simulink model "prueba_flujocarga_10_dic"  (R2015a)
settings: Solver=ode45  StartTime=0.0  StopTime=0.32  RelTol=1e-3
libraries: powerlib x31, powerlib_meascontrol x1
settings Model: Creator=USUARIO  LastModifiedBy=USUARIO

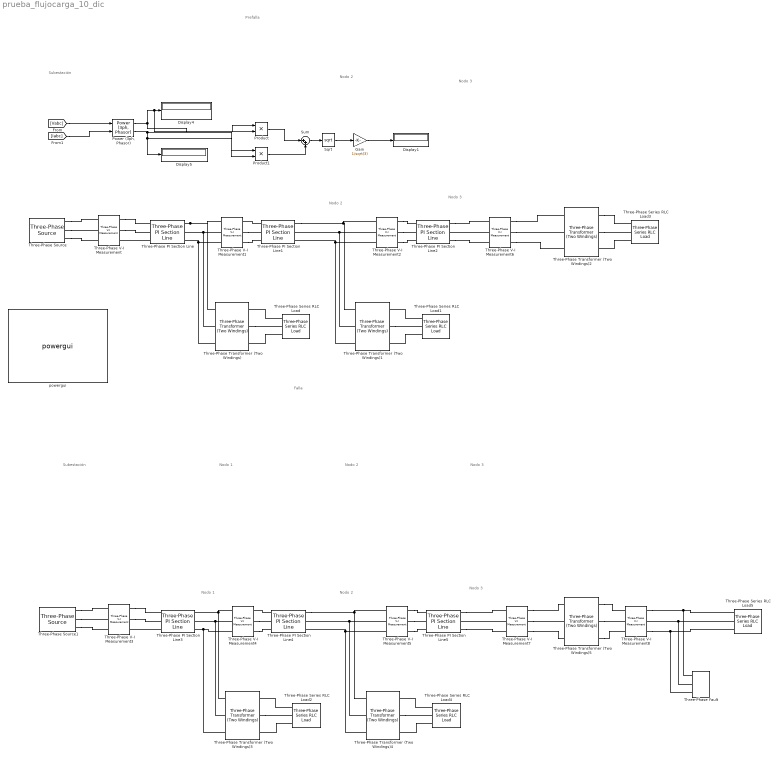
== system prueba_flujocarga_10_dic ==
  note: Falla
  note: Prefalla
  note: Nodo 2
  note: Subestación
  note: Nodo 2
  note: Nodo 1
  note: Nodo 1
  note: Nodo 2
  note: Subestación
  note: Nodo 2
  note: Nodo 3
  note: Nodo 3
  note: Nodo 3
  note: Nodo 3
  Display1 : Display
  Display4 : Display
  Display5 : Display
  Gain : Gain  Gain=1/sqrt(3)
  "Power (3ph, Phasor)" : powerlib_meascontrol/Measurements/Power (3ph, Phasor)
  Product : Product
  Product1 : Product
  Sqrt : Sqrt  SaturateOnIntegerOverflow=on
  Sum : Sum  Inputs=|++
  Three-Phase PI Section Line : powerlib/Elements/Three-Phase PI Section Line  LConnTagsString=a|b|c  RConnTagsString=A|B|C  Frequency=60  Resistances=[ 0.01273 0.3864]  Inductances="[ 0.9337e-3  4.1264e-3]"  Capacitances=[12.74e-9 7.751e-9]  Length=2
  Three-Phase PI Section Line1 : powerlib/Elements/Three-Phase PI Section Line  LConnTagsString=a|b|c  RConnTagsString=A|B|C  Frequency=60  Resistances=[ 0.01273 0.3864]  Inductances="[ 0.9337e-3  4.1264e-3]"  Capacitances=[12.74e-9 7.751e-9]  Length=1
  Three-Phase PI Section Line2 : powerlib/Elements/Three-Phase PI Section Line  LConnTagsString=a|b|c  RConnTagsString=A|B|C  Frequency=60  Resistances=[ 0.01273 0.3864]  Inductances="[ 0.9337e-3  4.1264e-3]"  Capacitances=[12.74e-9 7.751e-9]  Length=1.5
  Three-Phase PI Section Line3 : powerlib/Elements/Three-Phase PI Section Line  LConnTagsString=a|b|c  RConnTagsString=A|B|C  Frequency=60  Resistances=[ 0.01273 0.3864]  Inductances="[ 0.9337e-3  4.1264e-3]"  Capacitances=[12.74e-9 7.751e-9]  Length=2
  Three-Phase PI Section Line4 : powerlib/Elements/Three-Phase PI Section Line  LConnTagsString=a|b|c  RConnTagsString=A|B|C  Frequency=60  Resistances=[ 0.01273 0.3864]  Inductances="[ 0.9337e-3  4.1264e-3]"  Capacitances=[12.74e-9 7.751e-9]  Length=1
  Three-Phase PI Section Line5 : powerlib/Elements/Three-Phase PI Section Line  LConnTagsString=a|b|c  RConnTagsString=A|B|C  Frequency=60  Resistances=[ 0.01273 0.3864]  Inductances="[ 0.9337e-3  4.1264e-3]"  Capacitances=[12.74e-9 7.751e-9]  Length=1.5
  Three-Phase Series RLC Load{,1..5} (6 alike) : powerlib/Elements/Three-Phase Series RLC Load  LConnTagsString=A|B|C  Configuration=Y (grounded)  NominalVoltage=13800  NominalFrequency=60  ActivePower=10e3  InductivePower=100  CapacitivePower=100  Measurements=None  LoadType=constant Z
  Three-Phase Transformer (Two Windings) : powerlib/Elements/Three-Phase Transformer (Two Windings)  Winding1Connection=Yg  Winding2Connection=Yg  CoreType=Three single-phase transformers  SetSaturation=off  Hysteresis=off  DataFile='hysteresis'  SetInitialFlux=off  Measurements=None  UNITS=pu  NominalPower=[ 250e6 , 60 ]  Winding1=[ 115e3 , 0.002 , 0.08 ]  Winding2=[ 13.8e3 , 0.002 , 0.08 ]  Rm=500  Lm=500  L0=0.5  Saturation=[ 0,0 ; 0.0024,1.2 ; 1.0,1.52 ]  InitialFluxes=[ 0.8 , -0.8 , 0.7 ]  MoreParameters=off  BreakLoop=off  DataType=off  TransfoNumber=1
  Three-Phase Transformer (Two Windings){1..2,4..5} (4 alike) : powerlib/Elements/Three-Phase Transformer (Two Windings)  Winding1Connection=Yg  Winding2Connection=Yg  CoreType=Three single-phase transformers  SetSaturation=off  Hysteresis=off  DataFile='hysteresis'  SetInitialFlux=off  Measurements=None  UNITS=pu  NominalPower=[ 150e6 , 60 ]  Winding1=[ 115e3 , 0.002 , 0.08 ]  Winding2=[ 13.8e3 , 0.002 , 0.08 ]  Rm=500  Lm=500  L0=0.5  Saturation=[ 0,0 ; 0.0024,1.2 ; 1.0,1.52 ]  InitialFluxes=[ 0.8 , -0.8 , 0.7 ]  MoreParameters=off  BreakLoop=off  DataType=off  TransfoNumber=1
  Three-Phase Transformer (Two Windings)3 : powerlib/Elements/Three-Phase Transformer (Two Windings)  Winding1Connection=Yg  Winding2Connection=Yg  CoreType=Three single-phase transformers  SetSaturation=off  Hysteresis=off  DataFile='hysteresis'  SetInitialFlux=off  Measurements=None  UNITS=pu  NominalPower=[ 250e6 , 60 ]  Winding1=[ 115e3 , 0.002 , 0.08 ]  Winding2=[ 13.8e3 , 0.002 , 0.08 ]  Rm=500  Lm=500  L0=0.5  Saturation=[ 0,0 ; 0.0024,1.2 ; 1.0,1.52 ]  InitialFluxes=[ 0.8 , -0.8 , 0.7 ]  MoreParameters=off  BreakLoop=off  DataType=off  TransfoNumber=1
  Three-Phase V-I Measurement : powerlib/Measurements/Three-Phase V-I Measurement  VoltageMeasurement=phase-to-phase  SetLabelV=on  LabelV=Vabc  Vpu=off  VpuLL=off  CurrentMeasurement=yes  SetLabelI=on  LabelI=Iabc  Ipu=off  Pbase=100e6  Vbase=500e3  OutputType=Complex  PhasorSimulation=on  PSBequivalent=0
  Three-Phase V-I Measurement1 : powerlib/Measurements/Three-Phase V-I Measurement  VoltageMeasurement=phase-to-phase  SetLabelV=on  LabelV=Vabc1  Vpu=off  VpuLL=off  CurrentMeasurement=yes  SetLabelI=on  LabelI=Iabc1  Ipu=off  Pbase=100e6  Vbase=500e3  OutputType=Complex  PhasorSimulation=on  PSBequivalent=0
  Three-Phase V-I Measurement2 : powerlib/Measurements/Three-Phase V-I Measurement  VoltageMeasurement=phase-to-phase  SetLabelV=on  LabelV=Vabc2  Vpu=off  VpuLL=off  CurrentMeasurement=yes  SetLabelI=on  LabelI=Iabc2  Ipu=off  Pbase=100e6  Vbase=500e3  OutputType=Complex  PhasorSimulation=on  PSBequivalent=0
  Three-Phase V-I Measurement3 : powerlib/Measurements/Three-Phase V-I Measurement  VoltageMeasurement=phase-to-phase  SetLabelV=on  LabelV=Vabcs  Vpu=off  VpuLL=off  CurrentMeasurement=yes  SetLabelI=on  LabelI=Iabcs  Ipu=off  Pbase=100e6  Vbase=500e3  OutputType=Complex  PhasorSimulation=on  PSBequivalent=0
  Three-Phase V-I Measurement4 : powerlib/Measurements/Three-Phase V-I Measurement  VoltageMeasurement=phase-to-phase  SetLabelV=on  LabelV=Vabcn1  Vpu=off  VpuLL=off  CurrentMeasurement=yes  SetLabelI=on  LabelI=Iabcn1  Ipu=off  Pbase=100e6  Vbase=500e3  OutputType=Complex  PhasorSimulation=on  PSBequivalent=0
  Three-Phase V-I Measurement5 : powerlib/Measurements/Three-Phase V-I Measurement  VoltageMeasurement=phase-to-phase  SetLabelV=on  LabelV=Vabcn2  Vpu=off  VpuLL=off  CurrentMeasurement=yes  SetLabelI=on  LabelI=Iabcn2  Ipu=off  Pbase=100e6  Vbase=500e3  OutputType=Complex  PhasorSimulation=on  PSBequivalent=0
  Three-Phase V-I Measurement6 : powerlib/Measurements/Three-Phase V-I Measurement  VoltageMeasurement=phase-to-phase  SetLabelV=on  LabelV=Vabc3  Vpu=off  VpuLL=off  CurrentMeasurement=yes  SetLabelI=on  LabelI=Iabc3  Ipu=off  Pbase=100e6  Vbase=500e3  OutputType=Complex  PhasorSimulation=on  PSBequivalent=0
  Three-Phase V-I Measurement7 : powerlib/Measurements/Three-Phase V-I Measurement  VoltageMeasurement=phase-to-phase  SetLabelV=on  LabelV=Vabcn3  Vpu=off  VpuLL=off  CurrentMeasurement=yes  SetLabelI=on  LabelI=Iabcn3  Ipu=off  Pbase=100e6  Vbase=500e3  OutputType=Complex  PhasorSimulation=on  PSBequivalent=0
  Three-Phase V-I Measurement8 : powerlib/Measurements/Three-Phase V-I Measurement  VoltageMeasurement=phase-to-phase  SetLabelV=on  LabelV=Vabcn33  Vpu=off  VpuLL=off  CurrentMeasurement=yes  SetLabelI=on  LabelI=Iabcn33  Ipu=off  Pbase=100e6  Vbase=500e3  OutputType=Complex  PhasorSimulation=on  PSBequivalent=0
  Three-Phase Fault : powerlib/Elements/Three-Phase Fault  InitialStates=0  FaultA=on  FaultB=off  FaultC=off  GroundFault=on  SwitchTimes="[0.05  0.30]"  External=off  SwitchStatus=NaN  FaultResistance=0.001  GroundResistance=1  SnubberResistance=1e6  SnubberCapacitance=inf  Measurements=Fault currents
  Three-Phase Source : powerlib/Electrical Sources/Three-Phase Source  Voltage=115e3  PhaseAngle=0  Frequency=60  InternalConnection=Yg  SpecifyImpedance=on  Resistance=0.8929  Inductance=16.58e-3  ShortCircuitLevel=100e6  BaseVoltage=115e3  XRratio=7  BusType=swing  Pref=0  Qref=0  Qmin=-inf  Qmax=inf
  Three-Phase Source1 : powerlib/Electrical Sources/Three-Phase Source  Voltage=115e3  PhaseAngle=0  Frequency=60  InternalConnection=Yg  SpecifyImpedance=on  Resistance=0.8929  Inductance=16.58e-3  ShortCircuitLevel=100e6  BaseVoltage=115e3  XRratio=7  BusType=swing  Pref=0  Qref=0  Qmin=-inf  Qmax=inf
  powergui : powerlib/powergui  Priority=1  SimulationMode=Phasor  SolverType=Tustin  SampleTime=5.208333e-4  frequency=60  SPID=off  DisableSnubberDevices=off  DisableRonSwitches=off  DisableVfSwitches=off  SwTol=0  DisplayEquations=off  Interpol=off  methode=off  Ts=0  FunctionMessages=off  echomessages=off  HookPort=off  EnableUseOfTLC=off  x0status=blocks  frequencyindice=60  Pbase=100e6  ErrMax=1e-4  Iterations=50  UnitsV=kV  UnitsW=MW  buscounter=0  RestoreLinks=warning  ResistiveCurrentMeasurement=off  Frange=[0:2:500]  Ylog=off  Xlog=on  ShowGrid=off  save=off  variable=ZData  structure=0  ZoomFFT=off  StartTime=0.0  cycles=1  DisplayStyle=1  fundamental=60  FreqAxis=off  MaxFrequency=1000  frequencyindicesteady=1  RmsSteady=1  display=off
  wires:
  "Power (3ph, Phasor)"/1 -> Product/1, Display4/1, Product/2
  "Power (3ph, Phasor)"/2 -> Product1/1, Product1/2, Display5/1
  [Vabc] -> "Power (3ph, Phasor)"/1
  [Iabc] -> "Power (3ph, Phasor)"/2
  Gain/1 -> Display1/1
  Product/1 -> Sum/1
  Product1/1 -> Sum/2
  Sum/1 -> Sqrt/1
  Sqrt/1 -> Gain/1
  connections:
  Three-Phase PI Section Line/RConn1 -- Three-Phase Transformer (Two Windings)/LConn1 -- Three-Phase V-I Measurement1/LConn1
  Three-Phase Transformer (Two Windings)/LConn2 -- Three-Phase V-I Measurement1/LConn2 -- Three-Phase PI Section Line/RConn2
  Three-Phase Transformer (Two Windings)/LConn3 -- Three-Phase V-I Measurement1/LConn3 -- Three-Phase PI Section Line/RConn3
  Three-Phase PI Section Line1/RConn1 -- Three-Phase V-I Measurement2/LConn1 -- Three-Phase Transformer (Two Windings)1/LConn1
  Three-Phase Transformer (Two Windings)1/LConn2 -- Three-Phase V-I Measurement2/LConn2 -- Three-Phase PI Section Line1/RConn2
  Three-Phase Transformer (Two Windings)1/LConn3 -- Three-Phase V-I Measurement2/LConn3 -- Three-Phase PI Section Line1/RConn3
  Three-Phase V-I Measurement4/LConn1 -- Three-Phase Transformer (Two Windings)3/LConn1 -- Three-Phase PI Section Line3/RConn1
  Three-Phase V-I Measurement4/LConn2 -- Three-Phase Transformer (Two Windings)3/LConn2 -- Three-Phase PI Section Line3/RConn2
  Three-Phase V-I Measurement4/LConn3 -- Three-Phase Transformer (Two Windings)3/LConn3 -- Three-Phase PI Section Line3/RConn3
  Three-Phase PI Section Line4/RConn1 -- Three-Phase V-I Measurement5/LConn1 -- Three-Phase Transformer (Two Windings)4/LConn1
  Three-Phase Transformer (Two Windings)4/LConn2 -- Three-Phase V-I Measurement5/LConn2 -- Three-Phase PI Section Line4/RConn2
  Three-Phase Transformer (Two Windings)4/LConn3 -- Three-Phase V-I Measurement5/LConn3 -- Three-Phase PI Section Line4/RConn3
  Three-Phase Series RLC Load1/LConn3 -- Three-Phase Transformer (Two Windings)1/RConn3
  Three-Phase V-I Measurement/RConn1 -- Three-Phase PI Section Line/LConn1
  Three-Phase V-I Measurement/RConn2 -- Three-Phase PI Section Line/LConn2
  Three-Phase V-I Measurement2/RConn3 -- Three-Phase PI Section Line2/LConn3
  Three-Phase Series RLC Load/LConn1 -- Three-Phase Transformer (Two Windings)/RConn1
  Three-Phase V-I Measurement2/RConn2 -- Three-Phase PI Section Line2/LConn2
  Three-Phase PI Section Line1/LConn1 -- Three-Phase V-I Measurement1/RConn1
  Three-Phase V-I Measurement2/RConn1 -- Three-Phase PI Section Line2/LConn1
  Three-Phase V-I Measurement1/RConn2 -- Three-Phase PI Section Line1/LConn2
  Three-Phase Transformer (Two Windings)2/RConn1 -- Three-Phase Series RLC Load3/LConn1
  Three-Phase V-I Measurement1/RConn3 -- Three-Phase PI Section Line1/LConn3
  Three-Phase Transformer (Two Windings)1/RConn2 -- Three-Phase Series RLC Load1/LConn2
  Three-Phase Series RLC Load2/LConn3 -- Three-Phase Transformer (Two Windings)3/RConn3
  Three-Phase Source1/RConn2 -- Three-Phase V-I Measurement3/LConn2
  Three-Phase Series RLC Load4/LConn3 -- Three-Phase Transformer (Two Windings)4/RConn3
  Three-Phase Source1/RConn1 -- Three-Phase V-I Measurement3/LConn1
  Three-Phase PI Section Line3/LConn3 -- Three-Phase V-I Measurement3/RConn3
  Three-Phase Transformer (Two Windings)3/RConn2 -- Three-Phase Series RLC Load2/LConn2
  Three-Phase Transformer (Two Windings)2/RConn2 -- Three-Phase Series RLC Load3/LConn2
  Three-Phase Series RLC Load3/LConn3 -- Three-Phase Transformer (Two Windings)2/RConn3
  Three-Phase Source/RConn3 -- Three-Phase V-I Measurement/LConn3
  Three-Phase Series RLC Load1/LConn1 -- Three-Phase Transformer (Two Windings)1/RConn1
  Three-Phase Transformer (Two Windings)/RConn2 -- Three-Phase Series RLC Load/LConn2
  Three-Phase V-I Measurement5/RConn2 -- Three-Phase PI Section Line5/LConn2
  Three-Phase V-I Measurement5/RConn1 -- Three-Phase PI Section Line5/LConn1
  Three-Phase V-I Measurement5/RConn3 -- Three-Phase PI Section Line5/LConn3
  Three-Phase V-I Measurement4/RConn3 -- Three-Phase PI Section Line4/LConn3
  Three-Phase PI Section Line4/LConn1 -- Three-Phase V-I Measurement4/RConn1
  Three-Phase V-I Measurement4/RConn2 -- Three-Phase PI Section Line4/LConn2
  Three-Phase Transformer (Two Windings)4/RConn2 -- Three-Phase Series RLC Load4/LConn2
  Three-Phase Series RLC Load4/LConn1 -- Three-Phase Transformer (Two Windings)4/RConn1
  Three-Phase Series RLC Load2/LConn1 -- Three-Phase Transformer (Two Windings)3/RConn1
  Three-Phase V-I Measurement3/RConn2 -- Three-Phase PI Section Line3/LConn2
  Three-Phase V-I Measurement3/RConn1 -- Three-Phase PI Section Line3/LConn1
  Three-Phase Series RLC Load/LConn3 -- Three-Phase Transformer (Two Windings)/RConn3
  Three-Phase PI Section Line/LConn3 -- Three-Phase V-I Measurement/RConn3
  Three-Phase Source/RConn2 -- Three-Phase V-I Measurement/LConn2
  Three-Phase Source1/RConn3 -- Three-Phase V-I Measurement3/LConn3
  Three-Phase Source/RConn1 -- Three-Phase V-I Measurement/LConn1
  Three-Phase PI Section Line2/RConn1 -- Three-Phase V-I Measurement6/LConn1
  Three-Phase V-I Measurement6/LConn2 -- Three-Phase PI Section Line2/RConn2
  Three-Phase PI Section Line2/RConn3 -- Three-Phase V-I Measurement6/LConn3
  Three-Phase V-I Measurement6/RConn2 -- Three-Phase Transformer (Two Windings)2/LConn2
  Three-Phase V-I Measurement6/RConn1 -- Three-Phase Transformer (Two Windings)2/LConn1
  Three-Phase V-I Measurement6/RConn3 -- Three-Phase Transformer (Two Windings)2/LConn3
  Three-Phase PI Section Line5/RConn1 -- Three-Phase V-I Measurement7/LConn1
  Three-Phase V-I Measurement7/LConn2 -- Three-Phase PI Section Line5/RConn2
  Three-Phase PI Section Line5/RConn3 -- Three-Phase V-I Measurement7/LConn3
  Three-Phase V-I Measurement7/RConn2 -- Three-Phase Transformer (Two Windings)5/LConn2
  Three-Phase V-I Measurement7/RConn1 -- Three-Phase Transformer (Two Windings)5/LConn1
  Three-Phase V-I Measurement7/RConn3 -- Three-Phase Transformer (Two Windings)5/LConn3
  Three-Phase Transformer (Two Windings)5/RConn2 -- Three-Phase V-I Measurement8/LConn2
  Three-Phase Transformer (Two Windings)5/RConn3 -- Three-Phase V-I Measurement8/LConn3
  Three-Phase Transformer (Two Windings)5/RConn1 -- Three-Phase V-I Measurement8/LConn1
  Three-Phase V-I Measurement8/RConn1 -- Three-Phase Fault/LConn1 -- Three-Phase Series RLC Load5/LConn1
  Three-Phase Series RLC Load5/LConn2 -- Three-Phase Fault/LConn2 -- Three-Phase V-I Measurement8/RConn2
  Three-Phase V-I Measurement8/RConn3 -- Three-Phase Fault/LConn3 -- Three-Phase Series RLC Load5/LConn3
